simulink model "PID_sim"  (R2017b)
settings: Solver=ode45  StartTime=0.0  StopTime=endtime  FixedStep=T  RelTol=1e-3  EnableMultiTasking=on
values from neighbouring files (symbols this model uses):
  den_H = 1    [PID_config.m]
  Kd = 0.35    [PID_config.m]
  Ki = 0.005    [PID_config.m]
  Kn = 0    [PID_config.m]
  Kp = 7.5    [PID_config.m]
  num_H = 1    [PID_config.m]
  Psatmax = inf    [PID_config.m]
  Psatmin = -inf    [PID_config.m]
  T = 1 / fs    (= 0.0025)    [PID_config.m]
  Tdly = T/10    (= 0.00025)    [PID_config.m]
  Umax = inf    [PID_config.m]
  Umin = -inf    [PID_config.m]
  Vadc_max = inf    [PID_config.m]
  Vadc_min = -inf    [PID_config.m]
undefined symbols (not defined in the file or in its folder): den_G, num_G
libraries: simulink x3, DCL x1
settings Model: Creator=a0741273  LastModifiedBy=a0741273
settings DataIOCC: SaveFormat=Array  SignalLoggingSaveFormat=ModelDataLogs  SignalLogging=off
settings OptimizationCC: ExpressionDepthLimit=2147483647  InitFltsAndDblsToZero=on  LifeSpan=inf
settings DebuggingCC: SignalInfNanChecking=warning  SignalRangeChecking=warning  UnderspecifiedInitializationDetection=Classic  MergeDetectMultiDrivingBlocksExec=none  SolverPrmCheckMsg=warning  CheckMatrixSingularityMsg=warning  ParameterPrecisionLossMsg=none  FcnCallInpInsideContextMsg=warning  StateNameClashWarn=warning  SFUnexpectedBacktrackingDiag=warning  SFNoUnconditionalDefaultTransitionDiag=warning  SFExecutionAtInitializationDiag=none
settings HardwareCC: ProdBitPerPointer=32  ProdBitPerSizeT=32  ProdBitPerPtrDiffT=32  ProdLargestAtomicFloat=None  ProdIntDivRoundTo=Undefined  ProdEndianess=Unspecified  ProdWordSize=32  ProdHWDeviceType=32-bit Generic
settings ModelReferenceCC: PropagateSignalLabelsOutOfModel=off
settings CodeAppCC: StateflowObjectComments=on
settings GRTTargetCC: TargetLangStandard=C89/C90 (ANSI)  GeneratePreprocessorConditionals=Disable all  CombineOutputUpdateFcns=off  GRTInterface=on
settings ConfigComp: CovMetricSettings=dw  CovHtmlReporting=on  CovSaveCumulativeToWorkspaceVar=on  CovSaveSingleToWorkspaceVar=on  CovExternalEMLEnable=off  CovSFcnEnable=off

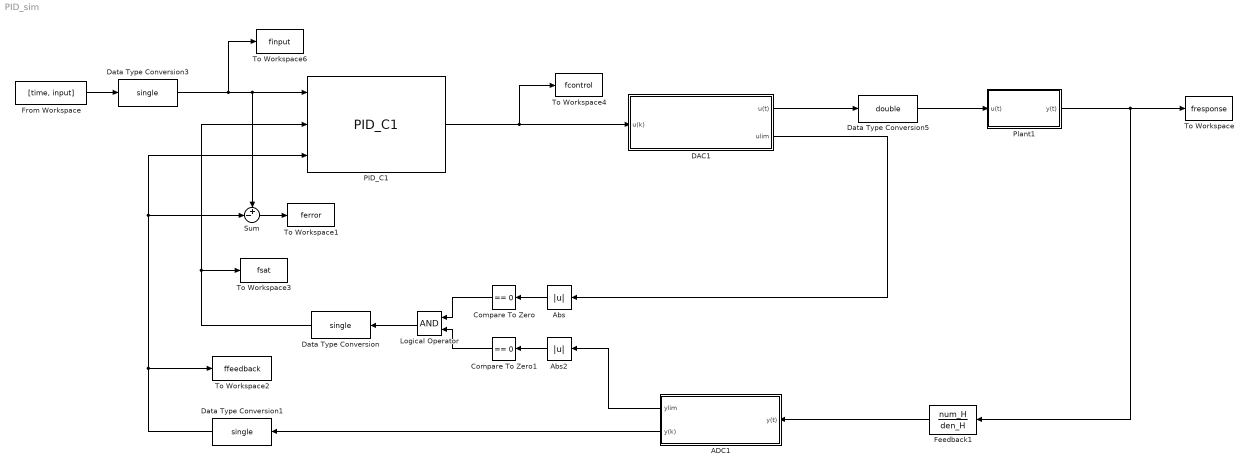
== system PID_sim ==
  ADC1 : Subsystem
  Abs : Abs
  Abs2 : Abs
  Compare To Zero : simulink/Logic and Bit Operations/Compare To Zero  relop===  OutDataTypeStr=uint8  ZeroCross=off
  Compare To Zero1 : simulink/Logic and Bit Operations/Compare To Zero  relop===  OutDataTypeStr=uint8  ZeroCross=off
  DAC1 : Subsystem
  Data Type Conversion : DataTypeConversion  OutDataTypeStr=single
  Data Type Conversion1 : DataTypeConversion  OutDataTypeStr=single  SaturateOnIntegerOverflow=on
  Data Type Conversion3 : DataTypeConversion  OutDataTypeStr=single  SaturateOnIntegerOverflow=on
  Data Type Conversion5 : DataTypeConversion  OutDataTypeStr=double
  Feedback1 : TransferFcn  Numerator=num_H  Denominator=den_H
  From Workspace : FromWorkspace  VariableName=[time, input]  SampleTime=T
  Logical Operator : Logic  AllPortsSameDT=off  OutDataTypeStr=boolean
  PID_C1 : DCL/PID_C1  Kp=Kp  Ki=Ki  Kd=Kd  Kr=Kr  fc=fc  Umax=Umax  Umin=Umin  T=T
  Plant1 : Subsystem
  Sum : Sum  Inputs=+-|
  To Workspace : ToWorkspace  VariableName=fresponse  SaveFormat=Timeseries  SampleTime=-1
  To Workspace1 : ToWorkspace  VariableName=ferror  SampleTime=-1
  To Workspace2 : ToWorkspace  VariableName=ffeedback  SampleTime=-1
  To Workspace3 : ToWorkspace  VariableName=fsat  SampleTime=-1
  To Workspace4 : ToWorkspace  VariableName=fcontrol  SampleTime=-1
  To Workspace6 : ToWorkspace  VariableName=finput  SampleTime=-1
  wires:
  From Workspace/1 -> Data Type Conversion3/1
  Abs/1 -> Compare To Zero/1
  Data Type Conversion1/1 -> PID_C1/3, Sum/2, To Workspace2/1
  Abs2/1 -> Compare To Zero1/1
  Compare To Zero1/1 -> Logical Operator/2
  Compare To Zero/1 -> Logical Operator/1
  Logical Operator/1 -> Data Type Conversion/1
  Data Type Conversion/1 -> To Workspace3/1, PID_C1/2
  ADC1/1(ylim) -> Abs2/1
  ADC1/2(y(k)) -> Data Type Conversion1/1
  PID_C1/1 -> To Workspace4/1, DAC1/1(u(k))
  DAC1/1(u(t)) -> Data Type Conversion5/1
  DAC1/2(ulim) -> Abs/1
  Data Type Conversion3/1 -> To Workspace6/1, PID_C1/1, Sum/1
  Plant1/1(y(t)) -> Feedback1/1, To Workspace/1
  Data Type Conversion5/1 -> Plant1/1(u(t))
  Feedback1/1 -> ADC1/1(y(t))
  Sum/1 -> To Workspace1/1

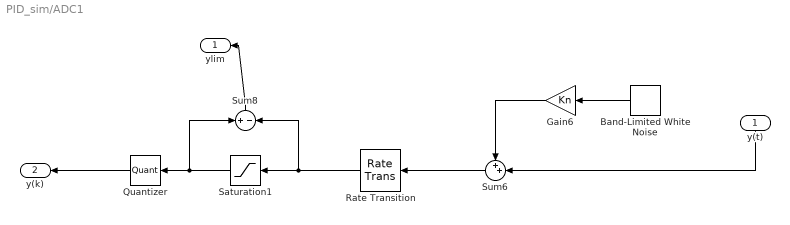
== system PID_sim/ADC1 ==
  y(t) : Inport
  Band-Limited White Noise : simulink/Sources/Band-Limited White Noise  Cov=[0.1]  Ts=T/100  seed=[23341]
  Gain6 : Gain  Gain=Kn
  Quantizer : Quantizer  QuantizationInterval=Qadc
  Rate Transition : RateTransition  OutPortSampleTime=T
  Saturation1 : Saturate  UpperLimit=Vadc_max  LowerLimit=Vadc_min
  Sum6 : Sum  Inputs=++|
  Sum8 : Sum  Inputs=+|-
  ylim : Outport
  y(k) : Outport  Port=2
  wires:
  Saturation1/1 -> Sum8/1, Quantizer/1
  Band-Limited White Noise/1 -> Gain6/1
  Sum6/1 -> Rate Transition/1
  Gain6/1 -> Sum6/1
  Rate Transition/1 -> Sum8/2, Saturation1/1
  Sum8/1 -> ylim/1
  Quantizer/1 -> y(k)/1
  y(t)/1 -> Sum6/2

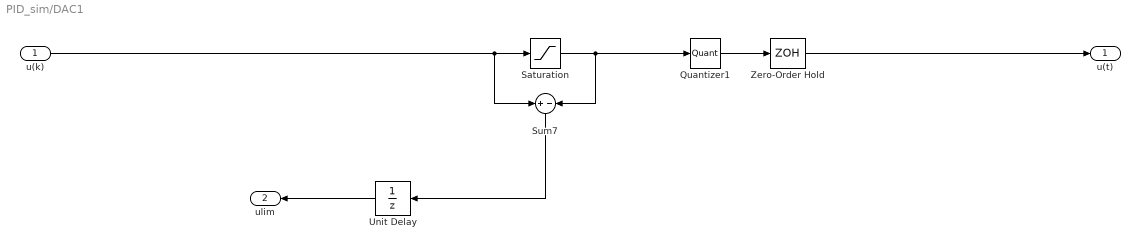
== system PID_sim/DAC1 ==
  u(k) : Inport
  Quantizer1 : Quantizer  QuantizationInterval=Qdac
  Saturation : Saturate  UpperLimit=Umax  LowerLimit=Umin
  Sum7 : Sum  Inputs=+|-
  Unit Delay : UnitDelay  SampleTime=-1
  Zero-Order Hold : ZeroOrderHold  SampleTime=-1
  u(t) : Outport
  ulim : Outport  Port=2
  wires:
  Zero-Order Hold/1 -> u(t)/1
  Quantizer1/1 -> Zero-Order Hold/1
  Sum7/1 -> Unit Delay/1
  Saturation/1 -> Quantizer1/1, Sum7/2
  u(k)/1 -> Sum7/1, Saturation/1
  Unit Delay/1 -> ulim/1

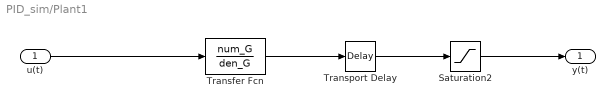
== system PID_sim/Plant1 ==
  u(t) : Inport
  Saturation2 : Saturate  UpperLimit=Psatmax  LowerLimit=Psatmin
  Transfer Fcn : TransferFcn  Numerator=num_G  Denominator=den_G
  Transport Delay : TransportDelay  DelayTime=Tdly  BufferSize=5120
  y(t) : Outport
  wires:
  Transfer Fcn/1 -> Transport Delay/1
  u(t)/1 -> Transfer Fcn/1
  Saturation2/1 -> y(t)/1
  Transport Delay/1 -> Saturation2/1
